simulink model "testing_platform_continuous_reaction_scaled_sensitivity"  (Simulink 7.9)
settings: Solver=ode45  StartTime=0.0  StopTime=10.0  RelTol=1e-3
values from neighbouring files (symbols this model uses):
  coeff = block.DialogPrm(1).Data    [continuous_reaction_model.m]    (also in continuous_reaction_model_scaled.m; continuous_reaction_model_scaled_sensitivity.m)
  x0 = block.DialogPrm(2).Data    [continuous_reaction_model.m]    (also in continuous_reaction_model_scaled.m; continuous_reaction_model_scaled_sensitivity.m)
settings Model: Creator=marco  LastModifiedBy=marco

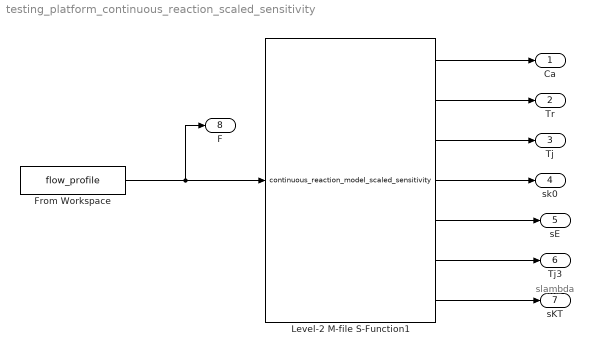
== system testing_platform_continuous_reaction_scaled_sensitivity ==
  note: slambda
  From Workspace : FromWorkspace  VariableName=flow_profile  SampleTime=0  Interpolate=off  OutputAfterFinalValue=Holding final value
  Level-2 M-file S-Function1 : M-S-Function  FunctionName=continuous_reaction_model_scaled_sensitivity  Parameters=coeff x0
  Ca : Outport
  Tr : Outport  Port=2
  Tj : Outport  Port=3
  sk0 : Outport  Port=4
  sE : Outport  Port=5
  Tj3 : Outport  Port=6
  sKT : Outport  Port=7
  F : Outport  Port=8
  wires:
  Level-2 M-file S-Function1/1 -> Ca/1
  Level-2 M-file S-Function1/2 -> Tr/1
  Level-2 M-file S-Function1/3 -> Tj/1
  From Workspace/1 -> Level-2 M-file S-Function1/1, F/1
  Level-2 M-file S-Function1/4 -> sk0/1
  Level-2 M-file S-Function1/5 -> sE/1
  Level-2 M-file S-Function1/6 -> Tj3/1
  Level-2 M-file S-Function1/7 -> sKT/1
